simulink model "model2b"  (R2017a)
settings: Solver=ode1  StartTime=0.0  StopTime=30  FixedStep=0.005  RelTol=1e-3  EnableMultiTasking=on
libraries: c6xlib x2, fricblocks x1
Description:
  | Real-Time Van der Pol Simulation
  | 
  | This demonstration shows a real-time version of the Simulink(R) Van der Pol
  | simulation demo. This model does not need any external signals, so it does
  | not need any data acquisition hardware or driver. This makes the model ideal
  | for first experiments with Real-Time Windows Target(TM), without need to
  | worry about proper I/O hardware configuration.
  | 
  | How to run this demo:
  | 
  |   1. Build the model using Tools -> Real-Time Workshop -> Build Model.
  |   2. Connect to the real-time code using Simulation -> Connect to target.
  |   3. Start the real-time execution using Simulation -> Start real-time code.
settings Model: SimulationMode=external  ExtModeTrigDuration=50000  Creator=Houska  LastModifiedBy=vjdixit2
settings DataIOCC: LimitDataPoints=on  SaveFormat=Array  SignalLoggingSaveFormat=ModelDataLogs  SignalLoggingName=logsOut
settings OptimizationCC: ExpressionDepthLimit=2147483647  InitFltsAndDblsToZero=on  EfficientMapNaN2IntZero=off
settings DebuggingCC: UnderspecifiedInitializationDetection=Classic  MergeDetectMultiDrivingBlocksExec=none  SignalResolutionControl=TryResolveAllWithWarning  FcnCallInpInsideContextMsg=warning  StateNameClashWarn=warning  SFUnexpectedBacktrackingDiag=warning  SFNoUnconditionalDefaultTransitionDiag=warning  SFExecutionAtInitializationDiag=none
settings ModelReferenceCC: PropagateSignalLabelsOutOfModel=off
settings RTWCC: SystemTargetFile=sldrt.tlc  TemplateMakefile=sldrt.tmf  Description=Simulink Desktop Real-Time  RTWCompilerOptimization=on
settings CodeAppCC: MaxIdLength=95
settings SimulinkDesktopRealTimeCC: TargetPreCompLibLocation=C:\MATLABR2017a\toolbox\sldrt\lib\win64  TargetLangStandard=C89/C90 (ANSI)  SupportVariableSizeSignals=off
settings ConfigComp: CovMetricSettings=dw  CovHtmlReporting=on  CovSaveCumulativeToWorkspaceVar=on  CovSaveSingleToWorkspaceVar=on  CovExternalEMLEnable=off  CovSFcnEnable=off

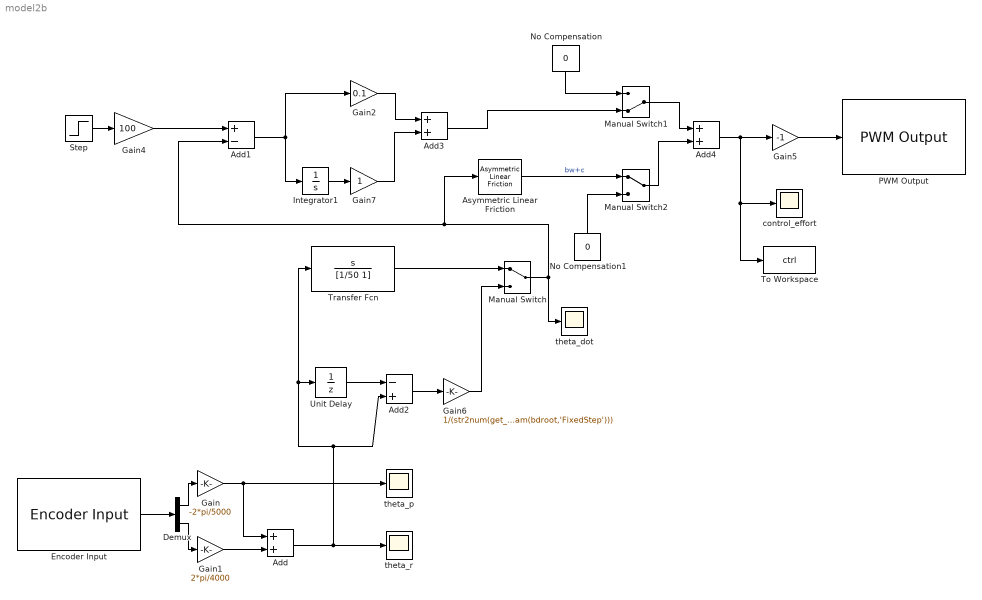
== system model2b ==
  Add : Sum
  Add1 : Sum  Inputs=+-
  Add2 : Sum  Inputs=-+
  Add3 : Sum
  Add4 : Sum
  Asymmetric Linear Friction : fricblocks/Asymmetric  Linear Friction  intercept1=0.605*(2/3)  intercept2=-.67*(2/3)  slope1=0.0126*(2/3)  slope2=0.0128*(2/3)
  Demux : Demux  Outputs=2
  Encoder Input : c6xlib/Encoder Input  baseAddr=0x378  channels=[0 1]  sampleTime=str2num(get_param(bdroot, 'FixedStep'))
  Gain : Gain  Gain=-2*pi/5000
  Gain1 : Gain  Gain=2*pi/4000
  Gain2 : Gain  Gain=0.1
  Gain4 : Gain  Gain=100
  Gain5 : Gain  Gain=-1
  Gain6 : Gain  Gain=1/(str2num(get_param(bdroot,'FixedStep')))
  Gain7 : Gain
  Integrator1 : Integrator
  Manual Switch : ManualSwitch
  Manual Switch1 : ManualSwitch  CurrentSetting=0
  Manual Switch2 : ManualSwitch
  No Compensation : Constant  Value=0
  No Compensation1 : Constant  Value=0
  PWM Output : c6xlib/PWM Output  baseAddr=0x378  channels=0  initialOutputs=0  finalOutputs=0  sampleTime=str2num(get_param(bdroot, 'FixedStep'))
  Step : Step  Time=0  SampleTime=0
  To Workspace : ToWorkspace  VariableName=ctrl  SampleTime=-1
  Transfer Fcn : TransferFcn  Numerator=[1 0]  Denominator=[1/50 1]
  Unit Delay : UnitDelay  SampleTime=-1
  "control_effort " : Scope
  "theta_dot " : Scope
  "theta_p " : Scope
  "theta_r " : Scope
  wires:
  Encoder Input/1 -> Demux/1
  Demux/1 -> Gain/1
  Demux/2 -> Gain1/1
  Gain/1 -> Add/1, "theta_p "/1
  Gain1/1 -> Add/2
  Add/1 -> "theta_r "/1, Transfer Fcn/1, Unit Delay/1, Add2/2
  Gain4/1 -> Add1/1
  Add1/1 -> Gain2/1, Integrator1/1
  Step/1 -> Gain4/1
  Gain5/1 -> PWM Output/1
  Unit Delay/1 -> Add2/1
  Add2/1 -> Gain6/1
  Transfer Fcn/1 -> Manual Switch/1
  Gain6/1 -> Manual Switch/2
  Manual Switch/1 -> "theta_dot "/1, Asymmetric Linear Friction/1, Add1/2
  Gain2/1 -> Add3/1
  Integrator1/1 -> Gain7/1
  Gain7/1 -> Add3/2
  Add4/1 -> To Workspace/1, "control_effort "/1, Gain5/1
  Add3/1 -> Manual Switch1/2
  Manual Switch1/1 -> Add4/1
  Asymmetric Linear Friction/1 -> Manual Switch2/1  "bw+c"
  Manual Switch2/1 -> Add4/2
  No Compensation/1 -> Manual Switch1/1
  No Compensation1/1 -> Manual Switch2/2
